simulink model "arduino_encoder_inc"  (R2023b)
settings: Solver=FixedStepDiscrete  StartTime=0.0  StopTime=inf  FixedStep=0.005  RelTol=1e-3  EnableMultiTasking=on
libraries: arduinolib x2, simulink x1
settings Model: ExtModeTrigDuration=2  Creator=yoany  LastModifiedBy=yoany
settings OptimizationCC: DefaultUnderspecifiedDataType=single  EnhancedBackFolding=on  PassReuseOutputArgsAs=Individual arguments  ZeroExternalMemoryAtStartup=off  ZeroInternalMemoryAtStartup=off  MaxStackSize=64  OptimizeBlockOrder=speed  DifferentSizesBufferReuse=on  OptimizationCustomize=off  EfficientTunableParamExpr=on
settings DebuggingCC: ParameterTunabilityLossMsg=error
settings HardwareCC: ProdBitPerInt=16  ProdBitPerPointer=16  ProdBitPerSizeT=16  ProdBitPerPtrDiffT=16  ProdLargestAtomicFloat=None  ProdWordSize=8  ProdHWDeviceType=Atmel->AVR  UseEmbeddedCoderFeatures=off
settings SFSimCC: MATLABDynamicMemAlloc=off
settings RTWCC: Description=Embedded Coder  SystemTargetFile=ert.tlc  HardwareBoard=Arduino Uno  TemplateMakefile=ert_default_tmf  Toolchain=Arduino AVR  BuildConfiguration=Faster Runs
settings CodeAppCC: ForceParamTrailComments=on  IgnoreCustomStorageClasses=off  OperatorAnnotations=on  SimulinkDataObjDesc=on  SFDataObjDesc=on  InsertBlockDesc=on
settings ERTTargetCC: SupportContinuousTime=on  SupportNonInlinedSFcns=on  SupportVariableSizeSignals=on  ExtModeTransport=3  ExtModeStaticAlloc=on  ExtModeAutomaticAllocSize=off  ExtModeStaticAllocSize=250  ExtModeMexFile=ext_xcp  ExtModeIntrfLevel=Level2 - Open

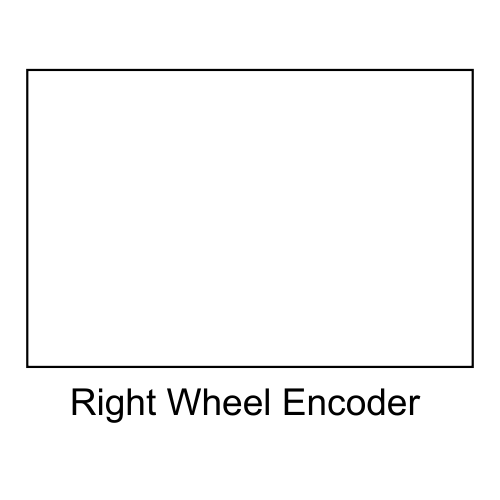
[thumbnail: Simulink's stored preview of the top-level diagram]
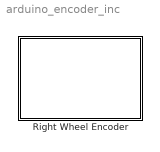
== system arduino_encoder_inc ==
  "Right Wheel Encoder " : Subsystem

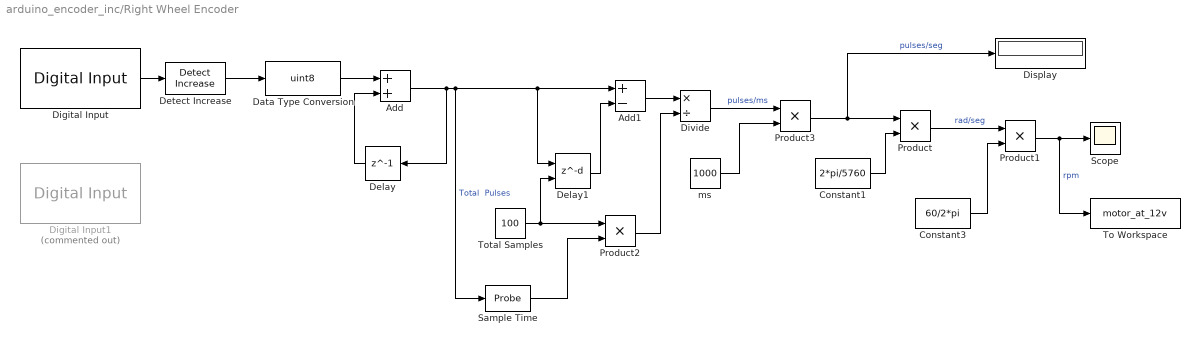
== system arduino_encoder_inc/Right Wheel Encoder  ==
  Add : Sum
  Add1 : Sum  Inputs=+-
  Constant1 : Constant  Value=2*pi/5760
  Constant3 : Constant  Value=60/2*pi  SampleTime=-1
  Data Type Conversion : DataTypeConversion  OutDataTypeStr=uint8  SaturateOnIntegerOverflow=off  RndMeth=Floor
  Delay : Delay  DelayLength=1
  Delay1 : Delay  DelayLengthSource=Input port  DelayLength=100
      settings: InputPortMap=u0,p1
  Detect Increase : simulink/Logic and Bit Operations/Detect Increase  vinit=0.0  OutDataTypeStr=boolean
  Digital Input : arduinolib/Digital Input  pinNumber=10  mode=Default  Direction=input  SampleTime=-1  blockPlatform=arduino
  Digital Input1 : arduinolib/Digital Input  Commented=on  pinNumber=11  mode=Default  Direction=input  SampleTime=0.001  blockPlatform=arduino
  Display : Display
  Divide : Product  Inputs=*/
  Product{,1..3} (4 alike) : Product
  Sample Time : Probe  ProbeWidth=off  ProbeComplexSignal=off
  Scope : Scope
  To Workspace : ToWorkspace  VariableName=motor_at_12v  SampleTime=-1
  Total Samples : Constant  Value=100  SampleTime=-1
  ms : Constant  Value=1000  SampleTime=-1
  wires:
  Delay/1 -> Add/2
  Add/1 -> Sample Time/1, Add1/1, Delay1/1, Delay/1  "Total  Pulses"
  Add1/1 -> Divide/1
  Delay1/1 -> Add1/2
  Digital Input/1 -> Detect Increase/1
  Detect Increase/1 -> Data Type Conversion/1
  Data Type Conversion/1 -> Add/1
  Constant1/1 -> Product/2
  Constant3/1 -> Product1/2
  Product/1 -> Product1/1  "rad/seg"
  Product1/1 -> To Workspace/1, Scope/1  "rpm"
  Total Samples/1 -> Product2/1, Delay1/2
  Sample Time/1 -> Product2/2
  Product2/1 -> Divide/2
  ms/1 -> Product3/2
  Divide/1 -> Product3/1  "pulses/ms"
  Product3/1 -> Display/1, Product/1  "pulses/seg"
